simulink model "LinearModelDevelopment_Example"  (R2015a)
settings: Solver=ode45  StartTime=0.0  StopTime=50  RelTol=1e-3
InitFcn:
  | Suspension_Parameters_2021
undefined symbols (not defined in the file): bs, Initial, ks, kt, mb, mw
settings Model: Creator=user  LastModifiedBy=user

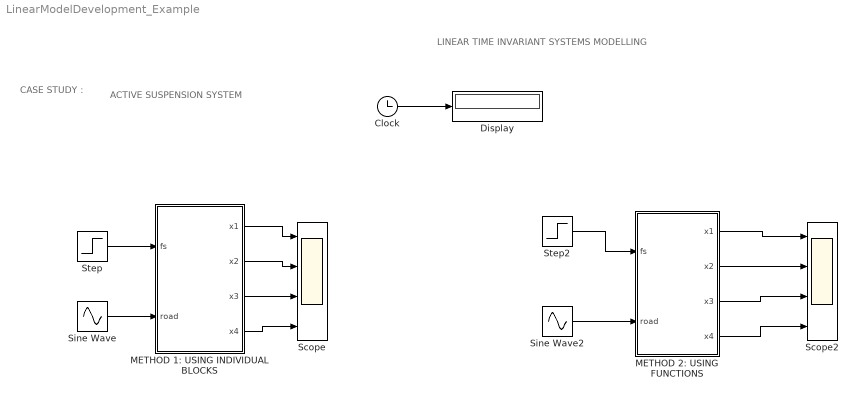
== system LinearModelDevelopment_Example ==
  note: ACTIVE SUSPENSION SYSTEM
  note: CASE STUDY :
  note: LINEAR TIME INVARIANT SYSTEMS MODELLING
  Clock : Clock
  Display : Display
  METHOD 1: USING INDIVIDUAL BLOCKS : Subsystem
  METHOD 2: USING FUNCTIONS : Subsystem
  Scope : Scope  NumInputPorts=4
      settings: YMin=-5~-5~-5~-5  YMax=5~5~5~5
  Scope2 : Scope  NumInputPorts=4
      settings: YMin=-5~-5~-5~-5  YMax=5~5~5~5  SaveName=ScopeData2
  Sine Wave : Sin  Amplitude=0.01  SampleTime=0
  Sine Wave2 : Sin  Amplitude=0.01  SampleTime=0
  Step : Step  SampleTime=0
  Step2 : Step  SampleTime=0
  wires:
  METHOD 1: USING INDIVIDUAL BLOCKS/1(x1) -> Scope/1
  METHOD 1: USING INDIVIDUAL BLOCKS/2(x2) -> Scope/2
  METHOD 1: USING INDIVIDUAL BLOCKS/3(x3) -> Scope/3
  METHOD 1: USING INDIVIDUAL BLOCKS/4(x4) -> Scope/4
  Step/1 -> METHOD 1: USING INDIVIDUAL BLOCKS/1(fs)
  Sine Wave/1 -> METHOD 1: USING INDIVIDUAL BLOCKS/2(road)
  Clock/1 -> Display/1
  Step2/1 -> METHOD 2: USING FUNCTIONS/1(fs)
  Sine Wave2/1 -> METHOD 2: USING FUNCTIONS/2(road)
  METHOD 2: USING FUNCTIONS/1(x1) -> Scope2/1
  METHOD 2: USING FUNCTIONS/2(x2) -> Scope2/2
  METHOD 2: USING FUNCTIONS/3(x3) -> Scope2/3
  METHOD 2: USING FUNCTIONS/4(x4) -> Scope2/4

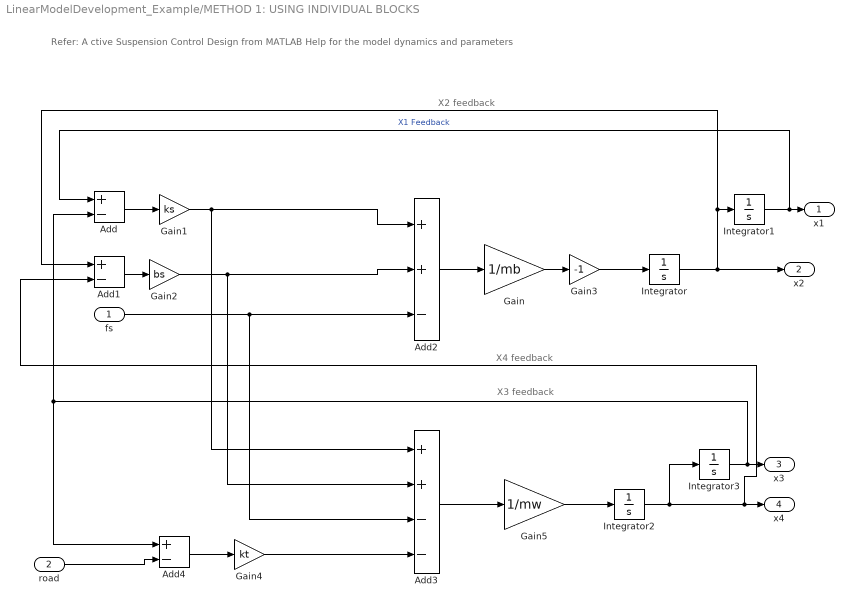
== system LinearModelDevelopment_Example/METHOD 1: USING INDIVIDUAL BLOCKS ==
  note: X2 feedback
  note: X3 feedback
  note: X4 feedback
  note: Refer: A ctive Suspension Control Design from MATLAB Help for the model dynamics and parameters
  fs : Inport
  road : Inport  Port=2
  Add : Sum  Inputs=+-
  Add1 : Sum  Inputs=+-
  Add2 : Sum  Inputs=++-
  Add3 : Sum  Inputs=++--
  Add4 : Sum  Inputs=+-
  Gain : Gain  Gain=1/mb
  Gain1 : Gain  Gain=ks
  Gain2 : Gain  Gain=bs
  Gain3 : Gain  Gain=-1
  Gain4 : Gain  Gain=kt
  Gain5 : Gain  Gain=1/mw
  Integrator : Integrator  InitialCondition=Initial.x2
  Integrator1 : Integrator  InitialCondition=Initial.x1
  Integrator2 : Integrator  InitialCondition=Initial.x4
  Integrator3 : Integrator  InitialCondition=Initial.x3
  x1 : Outport
  x2 : Outport  Port=2
  x3 : Outport  Port=3
  x4 : Outport  Port=4
  wires:
  Add/1 -> Gain1/1
  Add1/1 -> Gain2/1
  Integrator1/1 -> Add/1, x1/1  "X1 Feedback"
  Integrator3/1 -> x3/1, Add/2, Add4/1
  Integrator/1 -> Add1/1, Integrator1/1, x2/1
  Integrator2/1 -> Add1/2, x4/1, Integrator3/1
  Gain1/1 -> Add3/1, Add2/1
  Gain2/1 -> Add3/2, Add2/2
  fs/1 -> Add3/3, Add2/3
  Add2/1 -> Gain/1
  Gain/1 -> Gain3/1
  Gain3/1 -> Integrator/1
  road/1 -> Add4/2
  Add4/1 -> Gain4/1
  Gain4/1 -> Add3/4
  Add3/1 -> Gain5/1
  Gain5/1 -> Integrator2/1

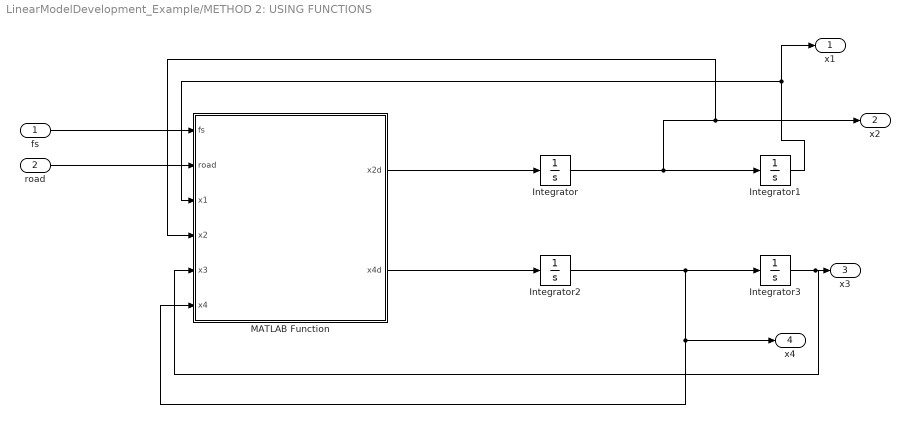
== system LinearModelDevelopment_Example/METHOD 2: USING FUNCTIONS ==
  fs : Inport
  road : Inport  Port=2
  Integrator : Integrator  InitialCondition=Initial.x2
  Integrator1 : Integrator  InitialCondition=Initial.x1
  Integrator2 : Integrator  InitialCondition=Initial.x4
  Integrator3 : Integrator  InitialCondition=Initial.x3
  MATLAB Function : MATLAB Function  TreatAsAtomicUnit=on
  x1 : Outport
  x2 : Outport  Port=2
  x3 : Outport  Port=3
  x4 : Outport  Port=4
  wires:
  MATLAB Function/1(x2d) -> Integrator/1
  Integrator/1 -> MATLAB Function/4(x2), x2/1, Integrator1/1
  MATLAB Function/2(x4d) -> Integrator2/1
  Integrator2/1 -> x4/1, MATLAB Function/6(x4), Integrator3/1
  Integrator1/1 -> MATLAB Function/3(x1), x1/1
  Integrator3/1 -> MATLAB Function/5(x3), x3/1
  road/1 -> MATLAB Function/2(road)
  fs/1 -> MATLAB Function/1(fs)

== matlab function LinearModelDevelopment_Example/METHOD 2: USING FUNCTIONS/MATLAB Function ==
  data: fs input; x2d output; road input; x4d output; x1 input; x2 input; x3 input; x4 input
function [x2d,x4d] = fcn(fs,road,x1,x2,x3,x4)
%#codegen

mb = 300;    % kg
mw = 60;     % kg
bs = 1000;   % N/m/s
ks = 16000 ; % N/m
kt = 190000; % N/m

x2d = -(1/mb)*(ks*(x1-x3)+ bs*(x2-x4)- fs);
x4d = (1/mw)*(ks*(x1-x3)+bs*(x2-x4)-kt*(x3-road)-fs);
